simulink library "approach"  (R2018b)
settings: Solver=VariableStepAuto  StartTime=0.0  StopTime=10.0  RelTol=1e-3
settings Model: Creator=chris  LastModifiedBy=chris

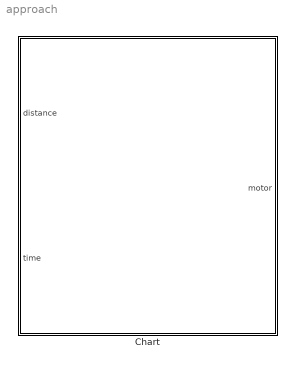
== system approach ==
  Chart : Stateflow chart  TreatAsAtomicUnit=on

== stateflow chart approach/Chart ==
  state Approach
    state Start
      entry: motor = 20
    state Wait
      entry: motor = 0
      entry: tstop = time + 5000
    state Exit
      entry: send(exitApproach)
    (default) -> Start
    Start -> Wait : [distance < stopDistance]
    Wait -> Exit : [time > tstop]
  state nextState
    % todo
    % go to next state
    % ??
  (default) -> Approach
  Approach -> nextState : exitApproach
  data: distance input; time input; motor output; tstop local; stopDistance constant double =20
  events: exitApproach local FUNCTION_CALL_EVENT
